simulink model "test"  (R2014a)
settings: Solver=ode45  StartTime=0.0  StopTime=10.0  RelTol=1e-3
libraries: dspbuff3 x2, dspmtrx3 x2
settings Model: Creator=root  LastModifiedBy=georg

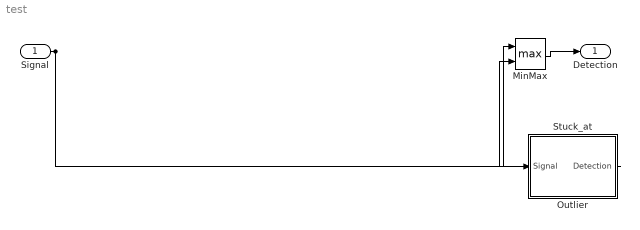
== system test ==
  Signal : Inport
  MinMax : MinMax  Function=max  Inputs=2
  Outlier : Subsystem
  Stuck_at : Subsystem
  Detection : Outport
  wires:
  MinMax/1 -> Detection/1
  Signal/1 -> Outlier/1(Signal), Stuck_at/1(Signal)
  Outlier/1(Detection) -> MinMax/1
  Stuck_at/1(Detection) -> MinMax/2

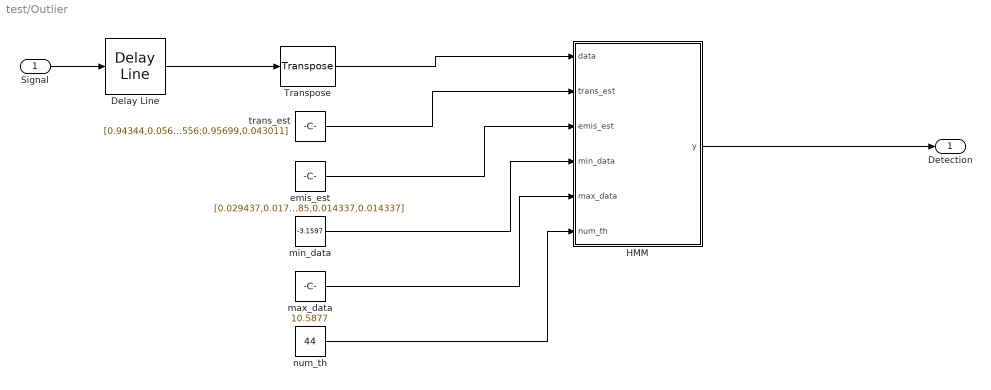
== system test/Outlier ==
  Signal : Inport
  Delay Line : dspbuff3/Delay Line  siz=1  ic=0  directfeed=off  enable_output=off  hold_output=off  TreatMby1Signals=One channel
  HMM : MATLAB Function  TreatAsAtomicUnit=on
  Transpose : dspmtrx3/Transpose  Hermitian=off  overflowFlag=off
  emis_est : Constant  Value=[0.029437,0.017366,0.024142,0.025837,0.030072,0.023931,0.02033,0.020542,0.019907,0.020754,0.033249,0.022872,0.029225,0.02986,0.021177,0.021177,0.020966,0.025201,0.030707,0.025201,0.019907,0.018848,0.017577,0.017789,0.019695,0.025625,0.018424,0.01906,0.020966,0.022236,0.024989,0.030496,0.038543,0.036425,0.025201,0.033037,0.031343,0.019695,0.015883,0.013342,0.016942,0.016095,0.0059297,0;0.0035842,0.0071685,0.02509,0.017921,0.017921,0.035842,0.02509,0.028674,0.032258,0.014337,0.010753,0.028674,0.021505,0.021505,0.032258,0.021505,0.035842,0.028674,0.028674,0.02509,0.032258,0.0071685,0.021505,0.017921,0.014337,0.014337,0.02509,0.014337,0.017921,0.032258,0.028674,0.014337,0.035842,0.021505,0.032258,0.032258,0.039427,0.032258,0.035842,0.014337,0.017921,0.0071685,0.014337,0.014337]
  max_data : Constant  Value=10.5877
  min_data : Constant  Value=-3.1597
  num_th : Constant  Value=44
  trans_est : Constant  Value=[0.94344,0.056556;0.95699,0.043011]
  Detection : Outport
  wires:
  Delay Line/1 -> Transpose/1
  Signal/1 -> Delay Line/1
  HMM/1(y) -> Detection/1
  num_th/1 -> HMM/6(num_th)
  min_data/1 -> HMM/4(min_data)
  trans_est/1 -> HMM/2(trans_est)
  max_data/1 -> HMM/5(max_data)
  Transpose/1 -> HMM/1(data)
  emis_est/1 -> HMM/3(emis_est)

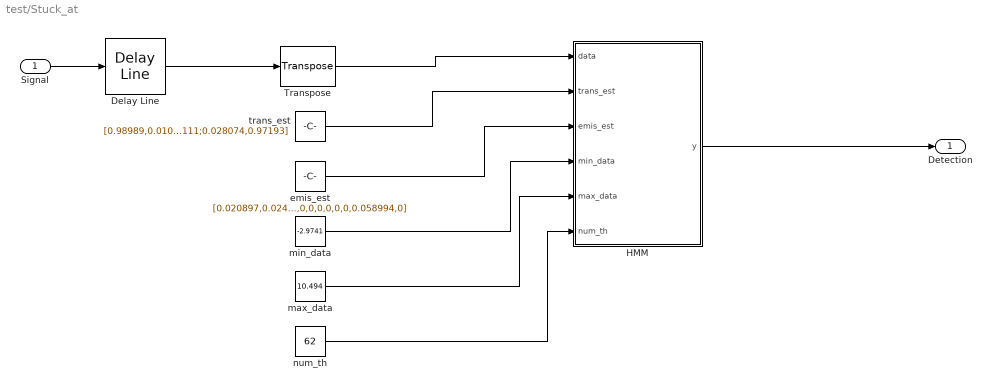
== system test/Stuck_at ==
  Signal : Inport
  Delay Line : dspbuff3/Delay Line  siz=6  ic=0  directfeed=off  enable_output=off  hold_output=off  TreatMby1Signals=One channel
  HMM : MATLAB Function  TreatAsAtomicUnit=on
  Transpose : dspmtrx3/Transpose  Hermitian=off  overflowFlag=off
  emis_est : Constant  Value=[0.020897,0.024267,0.014156,0.015167,0.012808,0.014156,0.015504,0.011459,0.026626,0.053927,0.036063,0.023256,0.020222,0.018874,0.018874,0.015167,0.014493,0.016178,0.026626,0.016515,0.012808,0.011122,0.011122,0.010785,0.008089,0.0091001,0.010448,0.0091001,0.0091001,0.010111,0.011122,0.013819,0.013482,0.012471,0.013482,0.012808,0.012471,0.012808,0.013145,0.013482,0.015167,0.016178,0.014493,0.015504,0.02393,0.02966,0.015504,0.033704,0.040445,0.045838,0.011459,0.014493,0.018874,0.0053927,0.0067408,0.0074149,0.011122,0.008426,0.0026963,0.0030334,0.0040445,0.0097742;0,0,0.020309,0,0.020309,0,0,0.020309,0.16151,0,0,0,0,0.30464,0.067698,0.00096712,0.020309,0,0,0.020309,0,0,0,0.020309,0.020309,0,0.020309,0.020309,0,0,0,0,0.020309,0.020309,0.020309,0,0,0.020309,0,0,0,0.034816,0,0,0,0,0,0.020309,0,0.040619,0,0.026112,0.020309,0,0,0,0,0,0,0,0.058994,0]
  max_data : Constant  Value=10.494
  min_data : Constant  Value=-2.9741
  num_th : Constant  Value=62
  trans_est : Constant  Value=[0.98989,0.010111;0.028074,0.97193]
  Detection : Outport
  wires:
  Delay Line/1 -> Transpose/1
  Signal/1 -> Delay Line/1
  HMM/1(y) -> Detection/1
  num_th/1 -> HMM/6(num_th)
  min_data/1 -> HMM/4(min_data)
  trans_est/1 -> HMM/2(trans_est)
  max_data/1 -> HMM/5(max_data)
  Transpose/1 -> HMM/1(data)
  emis_est/1 -> HMM/3(emis_est)

== matlab function test/Stuck_at/HMM ==
  data: data input; y output; trans_est input; emis_est input; min_data input; max_data input; num_th input
function y = fcn(data, trans_est, emis_est, min_data, max_data, num_th)
%#codegen
sd = size(data);
seq = ones(1,sd(1,2));

for i=1:num_th-1
    %get thresholds
    th = min_data + (max_data -min_data)*i/num_th;
    seq = seq + double(data >= th);
end

det = hmmviterbi(seq,trans_est,emis_est);
sdet = size(det);

y = det(1,sdet(1,2));
end

== matlab function test/Outlier/HMM ==
  data: data input; y output; trans_est input; emis_est input; min_data input; max_data input; num_th input
function y = fcn(data, trans_est, emis_est, min_data, max_data, num_th)
%#codegen
sd = size(data);
seq = ones(1,sd(1,2));

for i=1:num_th-1
    %get thresholds
    th = min_data + (max_data -min_data)*i/num_th;
    seq = seq + double(data >= th);
end

det = hmmviterbi(seq,trans_est,emis_est);
sdet = size(det);

y = det(1,sdet(1,2));
end
